simulink model "tensegrity_Val_like_sim_one_stage"  (R2022b)
settings: Solver=ode15s  StartTime=0.0  StopTime=10  MaxStep=0.001  RelTol=1e-3
InitFcn:
  | tensegrity_Val_like;
values from neighbouring files (symbols this model uses):
  a = 0.015    [parameters.m]
  A1 = [0.3, 0.3, 0.2]    [parameters_test_model.m]    (also in tensegrity_Val_like.m = [(G1+G2+G3)/3])
  bar_or_cable = 1    [parameters.m]
  bb = 100    [parameters.m]
  F1 = [pos1(1), pos1(2), pos1(3)]    [parameters.m]
  F2 = [pos1(1)+dist, pos1(2), pos1(3)]    [parameters.m]
  F3 = [pos1(1)+dist/2, pos1(2)+dist, pos1(3)]    [parameters.m]
  force_coefficient = -1    [parameters.m]
  kk = 5e4    (= 50000)    [parameters.m]
  l = [0.08 0.08 0.08 0.15]'    [parameters.m]
  lengths_0 = 0.9*lengths_0    [tensegrity_Val_like.m]
  lf = 0.05*ones(9, 1)    [parameters.m]
undefined symbols (not defined in the file or in its folder): X, Y, Z
libraries: nesl_utility x31, sm_lib x22
settings Model: Creator=zavrel  LastModifiedBy=zavrel

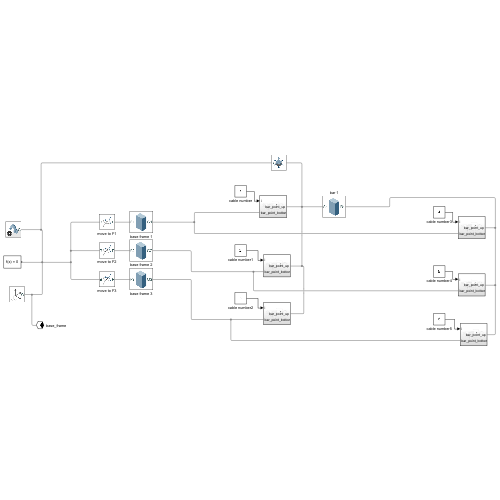
[thumbnail: Simulink's stored preview of the top-level diagram]
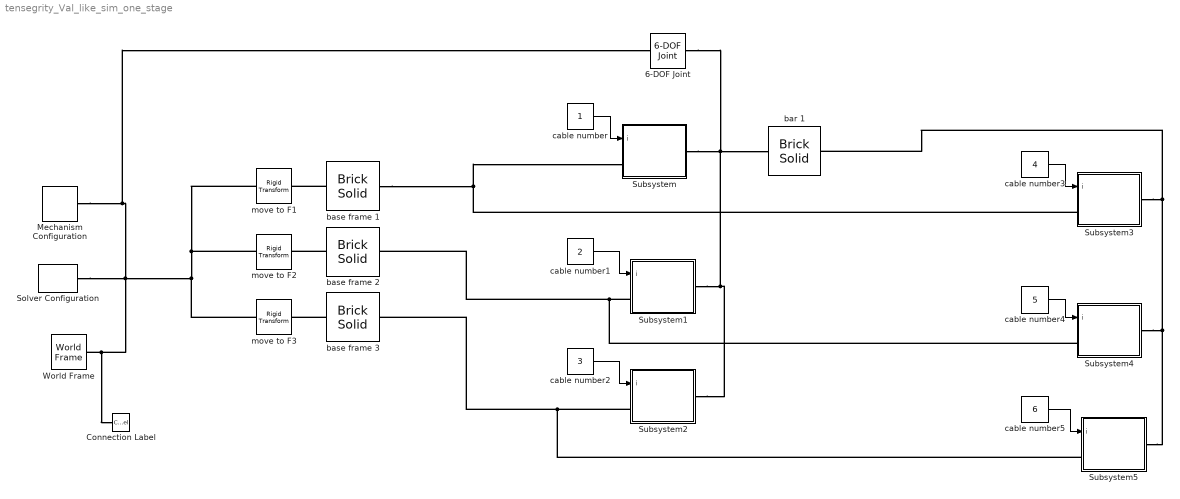
== system tensegrity_Val_like_sim_one_stage ==
  6-DOF Joint : sm_lib/Joints/6-DOF Joint  JointMode=Normal  SenseConstraintForce=off  SenseConstraintForceX=off  SenseConstraintForceY=off  SenseConstraintForceZ=off  SenseConstraintTorque=off  SenseConstraintTorqueX=off  SenseConstraintTorqueY=off  SenseConstraintTorqueZ=off  SenseTotalForce=off  SenseTotalForceX=off  SenseTotalForceY=off  SenseTotalForceZ=off  SenseTotalTorque=off  SenseTotalTorqueX=off  SenseTotalTorqueY=off  SenseTotalTorqueZ=off  CompositeWrenchDir=FollowerOnBase  CompositeWrenchFrame=BaseFrame  PxEquilibriumPosition=0  PxEquilibriumPositionUnits=m  PxSpringStiffness=0  PxSpringStiffnessUnits=N/m  PxDampingCoefficient=0  PxDampingCoefficientUnits=N/(m/s)  PxTorqueActuationMode=NoTorque  PxMotionActuationMode=ComputedMotion  PxSensePosition=off  PxSenseVelocity=off  PxSenseAcceleration=off  PxSenseTorqueForce=off  PxSenseLowerLimitTorqueForce=off  PxSenseUpperLimitTorqueForce=off  PxLowerLimitSpecify=off  PxLowerLimitBound=-1  PxLowerLimitBoundUnits=m  PxLowerLimitStiffness=1e6  PxLowerLimitStiffnessUnits=N/m  PxLowerLimitDamping=1e3  PxLowerLimitDampingUnits=N/(m/s)  PxLowerLimitTransitionRegionWidth=1e-4  PxLowerLimitTransitionRegionWidthUnits=m  PxUpperLimitSpecify=off  PxUpperLimitBound=1  PxUpperLimitBoundUnits=m  PxUpperLimitStiffness=1e6  PxUpperLimitStiffnessUnits=N/m  PxUpperLimitDamping=1e3  PxUpperLimitDampingUnits=N/(m/s)  PxUpperLimitTransitionRegionWidth=1e-4  PxUpperLimitTransitionRegionWidthUnits=m  PxPositionTargetSpecify=on  PxPositionTargetPriority=Low  PxPositionTargetValue=A1(1)  PxPositionTargetValueUnits=m  PxVelocityTargetSpecify=off  PxVelocityTargetPriority=High  PxVelocityTargetValue=0  PxVelocityTargetValueUnits=m/s  PyEquilibriumPosition=0  PyEquilibriumPositionUnits=m  PySpringStiffness=0  PySpringStiffnessUnits=N/m  PyDampingCoefficient=0  PyDampingCoefficientUnits=N/(m/s)  PyTorqueActuationMode=NoTorque  PyMotionActuationMode=ComputedMotion  PySensePosition=off  PySenseVelocity=off  PySenseAcceleration=off  PySenseTorqueForce=off  PySenseLowerLimitTorqueForce=off  PySenseUpperLimitTorqueForce=off  PyLowerLimitSpecify=off  PyLowerLimitBound=-1  PyLowerLimitBoundUnits=m  PyLowerLimitStiffness=1e6  PyLowerLimitStiffnessUnits=N/m  PyLowerLimitDamping=1e3  PyLowerLimitDampingUnits=N/(m/s)  PyLowerLimitTransitionRegionWidth=1e-4  PyLowerLimitTransitionRegionWidthUnits=m  PyUpperLimitSpecify=off  PyUpperLimitBound=1  PyUpperLimitBoundUnits=m  PyUpperLimitStiffness=1e6  PyUpperLimitStiffnessUnits=N/m  PyUpperLimitDamping=1e3  PyUpperLimitDampingUnits=N/(m/s)  PyUpperLimitTransitionRegionWidth=1e-4  PyUpperLimitTransitionRegionWidthUnits=m  PyPositionTargetSpecify=on  PyPositionTargetPriority=Low  PyPositionTargetValue=A1(2)  PyPositionTargetValueUnits=m  PyVelocityTargetSpecify=off  PyVelocityTargetPriority=High  PyVelocityTargetValue=0  PyVelocityTargetValueUnits=m/s  PzEquilibriumPosition=0  PzEquilibriumPositionUnits=m  PzSpringStiffness=0  PzSpringStiffnessUnits=N/m  PzDampingCoefficient=0  PzDampingCoefficientUnits=N/(m/s)  PzTorqueActuationMode=NoTorque  PzMotionActuationMode=ComputedMotion  PzSensePosition=off  PzSenseVelocity=off  PzSenseAcceleration=off  PzSenseTorqueForce=off  PzSenseLowerLimitTorqueForce=off  PzSenseUpperLimitTorqueForce=off  PzLowerLimitSpecify=off  PzLowerLimitBound=-1  PzLowerLimitBoundUnits=m  PzLowerLimitStiffness=1e6  PzLowerLimitStiffnessUnits=N/m  PzLowerLimitDamping=1e3  PzLowerLimitDampingUnits=N/(m/s)  PzLowerLimitTransitionRegionWidth=1e-4  PzLowerLimitTransitionRegionWidthUnits=m  PzUpperLimitSpecify=off  PzUpperLimitBound=1  PzUpperLimitBoundUnits=m  PzUpperLimitStiffness=1e6  PzUpperLimitStiffnessUnits=N/m  PzUpperLimitDamping=1e3  PzUpperLimitDampingUnits=N/(m/s)  PzUpperLimitTransitionRegionWidth=1e-4  PzUpperLimitTransitionRegionWidthUnits=m  PzPositionTargetSpecify=on  PzPositionTargetPriority=Low  PzPositionTargetValue=A1(3)  PzPositionTargetValueUnits=m  PzVelocityTargetSpecify=off  PzVelocityTargetPriority=High  PzVelocityTargetValue=0  PzVelocityTargetValueUnits=m/s  SphEqPosRotationMethod=None  SphEqPosRotationAngleUnits=deg  SphEqPosRotationStandardAxis=+Z  SphEqPosRotationAngle=0.0  SphEqPosRotationArbitraryAxis=[0 0 1]  SphEqPosFollAlignAxisA=+X  SphEqPosBaseAlignAxisA=+Y  SphEqPosFollAlignAxisB=+Y  SphEqPosBaseAlignAxisB=+Z  SphEqPosRotationSequenceAxes=FollowerAxes  SphEqPosRotationSequence=XYX  SphEqPosRotationSequenceAngles=[0 0 0]  SphEqPosRotationSequenceAnglesUnits=deg  SphEqPosRotationMatrix=[1 0 0; 0 1 0; 0 0 1]  SphEqPosQuaternion=[1 0 0 0]  SphSpringStiffness=0  SphSpringStiffnessUnits=N*m/deg  SphDampingCoefficient=0  SphDampingCoefficientUnits=N*m/(deg/s)  SphActuateTorqueX=off  SphActuateTorqueY=off  SphActuateTorqueZ=off  SphActuateTorque=off  SphTorqueActuationMode=NoTorque  SphMotionActuationMode=ComputedMotion  SphActuationFrame=BaseFrame  SphSensePosition=off  SphSenseVelocityX=off  SphSenseVelocityY=off  SphSenseVelocityZ=off  SphSenseVelocity=off  SphSenseAccelerationX=off  SphSenseAccelerationY=off  SphSenseAccelerationZ=off  SphSenseAcceleration=off  SphSenseTorqueX=off  SphSenseTorqueY=off  SphSenseTorqueZ=off  SphSenseTorqueForce=off  SphSenseLowerLimitTorqueMag=off  SphSenseUpperLimitTorqueMag=off  SphSensingFrame=BaseFrame  SphLowerLimitSpecify=off  SphLowerLimitBound=15  SphLowerLimitBoundUnits=deg  SphLowerLimitStiffness=1e4  SphLowerLimitStiffnessUnits=N*m/deg  SphLowerLimitDamping=10  SphLowerLimitDampingUnits=N*m/(deg/s)  SphLowerLimitTransitionRegionWidth=0.1  SphLowerLimitTransitionRegionWidthUnits=deg  SphUpperLimitSpecify=off  SphUpperLimitBound=45  SphUpperLimitBoundUnits=deg  SphUpperLimitStiffness=1e4  SphUpperLimitStiffnessUnits=N*m/deg  SphUpperLimitDamping=10  SphUpperLimitDampingUnits=N*m/(deg/s)  SphUpperLimitTransitionRegionWidth=0.1  SphUpperLimitTransitionRegionWidthUnits=deg  SphPositionTargetRotationMethod=None  SphPositionTargetRotationAngleUnits=deg  SphPositionTargetRotationStandardAxis=+Z  SphPositionTargetRotationAngle=0.0  SphPositionTargetRotationArbitraryAxis=[0 0 1]  SphPositionTargetFollAlignAxisA=+X  SphPositionTargetBaseAlignAxisA=+Y  SphPositionTargetFollAlignAxisB=+Y  SphPositionTargetBaseAlignAxisB=+Z  SphPositionTargetRotationSequenceAxes=FollowerAxes  SphPositionTargetRotationSequence=XYX  SphPositionTargetRotationSequenceAngles=[0 0 0]  SphPositionTargetRotationSequenceAnglesUnits=deg  SphPositionTargetRotationMatrix=[1 0 0; 0 1 0; 0 0 1]  SphPositionTargetQuaternion=[1 0 0 0]  SphPositionTargetSpecify=off  SphPositionTargetPriority=High  SphVelocityTargetValue=[0 0 0]  SphVelocityTargetValueUnits=deg/s  SphVelocityTargetSpecify=off  SphVelocityTargetPriority=High  SphVelocityTargetInFollowerFrame=on
  Connection Label : ConnectionLabel  Label=base_frame
  Mechanism Configuration : sm_lib/Utilities/Mechanism Configuration  UniformGravity=Constant  GravityVector=[0 0 -9.80665]  GravityUnits=m/s^2  LinearizationDelta=0.001  JointModeTransitionNonlinearIterations=2
  Solver Configuration : nesl_utility/Solver Configuration  PhysicalDomain=network_engine_domain  SubClassName=solver  LeftPortType=input  RightPortType=generic  Tones=[]  Harmonics=[]  SimulateNoise=off  Profile=off  UseLocalSampling=off  EnableSwitchedLinearOptims=on  FrequencyDomain=off  UseCCode=off  RelTol=0.001  AbsTol=0.001  MinStep=1e-09  ToWorkspace=off  RevertToSquareIcSolve=off  NumHomotopyIterations=100  PhasorMode=off  PhasorModeNumHarmonics=1  ConsistencySolver=NEWTON_XTOL_AFTER_FTOL  IndexReductionMethod=DerivativeReplacement  DoDC=off  ResidualTolerance=1e-09  ConsistencyTolSource=GLOBAL  ConsistencyAbsTol=0.001  ConsistencyRelTol=0.001  ConsistencyTolFactor=0.001  UseLocalSolver=off  LocalSolverChoice=NE_BACKWARD_EULER_ADVANCER  ResolveIndetEquations=on  FunctionEvalNumThread=1  LocalSolverSampleTime=0.001  DoFixedCost=off  MaxNonlinIter=3  MaxModeIter=2  ComputeImpulses=off  ImpulseIterations=2  LinearAlgebra=auto  LinearAlgebraNumThread=0  EquationFormulation=NE_TIME_EF  DelaysMemoryBudget=1024  AutomaticFiltering=on  FilteringTimeConstant=0.001  PartitionStorageMethod=AS_NEEDED  PartitionMemoryBudget=1024  PartitionMethod=ROBUST
  Subsystem : Subsystem
  Subsystem1 : Subsystem
  Subsystem2 : Subsystem
  Subsystem3 : Subsystem
  Subsystem4 : Subsystem
  Subsystem5 : Subsystem
  World Frame : sm_lib/Frames and Transforms/World Frame
  bar 1 : sm_lib/Body Elements/Brick Solid  GraphicAmbientColor=[0.15 0.15 0.15 1.0]  BasedOnType=Density  BrickDimensions=[a a l(1)]  BrickDimensionUnits=m  CenterOfMass=[0 0 0]  CenterOfMassUnits=m  GraphicDiffuseColor=[0.5 0.5 0.5]  Density=rho  DensityUnits=kg/m^3  DoExposeReferenceFrame=off  GraphicEmissiveColor=[0.0 0.0 0.0 1.0]  ExportEntireGeometry=off  SerializedFrames=<Frames><Frame><Id>Frame1</Id><Value><Name>A1</Name><Origin><Source>GeometricFeature</Source><FeatureName>-z surface</FeatureName></Origin><PrimaryAxis><DefinedDirection>+Z</DefinedDirection><Source>ReferenceFrame</Source><SourceDirection>+Z</SourceDirection><FeatureName></FeatureName></PrimaryAxis><SecondaryAxis><DefinedDirection>+X</DefinedDirection><Source>ReferenceFrame</Source><SourceDirection>+X</SourceDirection><FeatureName></FeatureName></SecondaryAxis></Value></Frame><Frame><Id>Frame2</Id><Value><Name>B1</Name><Origin><Source>GeometricFeature</Source><FeatureName>+z surface</FeatureName></Origin><PrimaryAxis><DefinedDirection>+Z</DefinedDirection><Source>ReferenceFrame</Source><SourceDirection>+Z</SourceDirection><FeatureName></FeatureName></PrimaryAxis><SecondaryAxis><DefinedDirection>+X</DefinedDirection><Source>ReferenceFrame</Source><SourceDirection>+X</SourceDirection><FeatureName></FeatureName></SecondaryAxis></Value></Frame></Frames>  MarkerShape=Sphere  MarkerSize=10  GraphicType=FromGeometry  InertiaType=CalculateFromGeometry  Mass=1  MassUnits=kg  MomentsOfInertia=[1 1 1]  MomentsOfInertiaUnits=kg*m^2  GraphicOpacity=1.0  ProductsOfInertia=[0 0 0]  ProductsOfInertiaUnits=kg*m^2  GraphicShininess=75  GraphicSpecularColor=[0.5 0.5 0.5 1.0]  GraphicVisPropType=SimpleVisualProperties
  base frame 1 : sm_lib/Body Elements/Brick Solid  GraphicAmbientColor=[0.15 0.15 0.15 1.0]  BasedOnType=Density  BrickDimensions=[a a lf(1)]  BrickDimensionUnits=m  CenterOfMass=[0 0 0]  CenterOfMassUnits=m  GraphicDiffuseColor=[0.5 0.5 0.5]  Density=rho  DensityUnits=kg/m^3  DoExposeReferenceFrame=off  GraphicEmissiveColor=[0.0 0.0 0.0 1.0]  ExportEntireGeometry=off  SerializedFrames=<Frames><Frame><Id>Frame1</Id><Value><Name>F1</Name><Origin><Source>GeometricFeature</Source><FeatureName>-z surface</FeatureName></Origin><PrimaryAxis><DefinedDirection>+Z</DefinedDirection><Source>ReferenceFrame</Source><SourceDirection>+Z</SourceDirection><FeatureName></FeatureName></PrimaryAxis><SecondaryAxis><DefinedDirection>+X</DefinedDirection><Source>ReferenceFrame</Source><SourceDirection>+X</SourceDirection><FeatureName></FeatureName></SecondaryAxis></Value></Frame><Frame><Id>Frame2</Id><Value><Name>G1</Name><Origin><Source>GeometricFeature</Source><FeatureName>+z surface</FeatureName></Origin><PrimaryAxis><DefinedDirection>+Z</DefinedDirection><Source>ReferenceFrame</Source><SourceDirection>+Z</SourceDirection><FeatureName></FeatureName></PrimaryAxis><SecondaryAxis><DefinedDirection>+X</DefinedDirection><Source>ReferenceFrame</Source><SourceDirection>+X</SourceDirection><FeatureName></FeatureName></SecondaryAxis></Value></Frame></Frames>  MarkerShape=Sphere  MarkerSize=10  GraphicType=FromGeometry  InertiaType=CalculateFromGeometry  Mass=1  MassUnits=kg  MomentsOfInertia=[1 1 1]  MomentsOfInertiaUnits=kg*m^2  GraphicOpacity=1.0  ProductsOfInertia=[0 0 0]  ProductsOfInertiaUnits=kg*m^2  GraphicShininess=75  GraphicSpecularColor=[0.5 0.5 0.5 1.0]  GraphicVisPropType=SimpleVisualProperties
  base frame 2 : sm_lib/Body Elements/Brick Solid  GraphicAmbientColor=[0.15 0.15 0.15 1.0]  BasedOnType=Density  BrickDimensions=[a a lf(2)]  BrickDimensionUnits=m  CenterOfMass=[0 0 0]  CenterOfMassUnits=m  GraphicDiffuseColor=[0.5 0.5 0.5]  Density=rho  DensityUnits=kg/m^3  DoExposeReferenceFrame=off  GraphicEmissiveColor=[0.0 0.0 0.0 1.0]  ExportEntireGeometry=off  SerializedFrames=<Frames><Frame><Id>Frame1</Id><Value><Name>F2</Name><Origin><Source>GeometricFeature</Source><FeatureName>-z surface</FeatureName></Origin><PrimaryAxis><DefinedDirection>+Z</DefinedDirection><Source>ReferenceFrame</Source><SourceDirection>+Z</SourceDirection><FeatureName></FeatureName></PrimaryAxis><SecondaryAxis><DefinedDirection>+X</DefinedDirection><Source>ReferenceFrame</Source><SourceDirection>+X</SourceDirection><FeatureName></FeatureName></SecondaryAxis></Value></Frame><Frame><Id>Frame2</Id><Value><Name>G2</Name><Origin><Source>GeometricFeature</Source><FeatureName>+z surface</FeatureName></Origin><PrimaryAxis><DefinedDirection>+Z</DefinedDirection><Source>ReferenceFrame</Source><SourceDirection>+Z</SourceDirection><FeatureName></FeatureName></PrimaryAxis><SecondaryAxis><DefinedDirection>+X</DefinedDirection><Source>ReferenceFrame</Source><SourceDirection>+X</SourceDirection><FeatureName></FeatureName></SecondaryAxis></Value></Frame></Frames>  MarkerShape=Sphere  MarkerSize=10  GraphicType=FromGeometry  InertiaType=CalculateFromGeometry  Mass=1  MassUnits=kg  MomentsOfInertia=[1 1 1]  MomentsOfInertiaUnits=kg*m^2  GraphicOpacity=1.0  ProductsOfInertia=[0 0 0]  ProductsOfInertiaUnits=kg*m^2  GraphicShininess=75  GraphicSpecularColor=[0.5 0.5 0.5 1.0]  GraphicVisPropType=SimpleVisualProperties
  base frame 3 : sm_lib/Body Elements/Brick Solid  GraphicAmbientColor=[0.15 0.15 0.15 1.0]  BasedOnType=Density  BrickDimensions=[a a lf(3)]  BrickDimensionUnits=m  CenterOfMass=[0 0 0]  CenterOfMassUnits=m  GraphicDiffuseColor=[0.5 0.5 0.5]  Density=rho  DensityUnits=kg/m^3  DoExposeReferenceFrame=off  GraphicEmissiveColor=[0.0 0.0 0.0 1.0]  ExportEntireGeometry=off  SerializedFrames=<Frames><Frame><Id>Frame1</Id><Value><Name>F3</Name><Origin><Source>GeometricFeature</Source><FeatureName>-z surface</FeatureName></Origin><PrimaryAxis><DefinedDirection>+Z</DefinedDirection><Source>ReferenceFrame</Source><SourceDirection>+Z</SourceDirection><FeatureName></FeatureName></PrimaryAxis><SecondaryAxis><DefinedDirection>+X</DefinedDirection><Source>ReferenceFrame</Source><SourceDirection>+X</SourceDirection><FeatureName></FeatureName></SecondaryAxis></Value></Frame><Frame><Id>Frame2</Id><Value><Name>G3</Name><Origin><Source>GeometricFeature</Source><FeatureName>+z surface</FeatureName></Origin><PrimaryAxis><DefinedDirection>+Z</DefinedDirection><Source>ReferenceFrame</Source><SourceDirection>+Z</SourceDirection><FeatureName></FeatureName></PrimaryAxis><SecondaryAxis><DefinedDirection>+X</DefinedDirection><Source>ReferenceFrame</Source><SourceDirection>+X</SourceDirection><FeatureName></FeatureName></SecondaryAxis></Value></Frame></Frames>  MarkerShape=Sphere  MarkerSize=10  GraphicType=FromGeometry  InertiaType=CalculateFromGeometry  Mass=1  MassUnits=kg  MomentsOfInertia=[1 1 1]  MomentsOfInertiaUnits=kg*m^2  GraphicOpacity=1.0  ProductsOfInertia=[0 0 0]  ProductsOfInertiaUnits=kg*m^2  GraphicShininess=75  GraphicSpecularColor=[0.5 0.5 0.5 1.0]  GraphicVisPropType=SimpleVisualProperties
  cable number : Constant
  cable number1 : Constant  Value=2
  cable number2 : Constant  Value=3
  cable number3 : Constant  Value=4
  cable number4 : Constant  Value=5
  cable number5 : Constant  Value=6
  move to F1 : sm_lib/Frames and Transforms/Rigid Transform  TranslationMethod=Cartesian  TranslationStandardOffset=0  TranslationLengthUnit=m  TranslationStandardAxis=+Z  TranslationCartesianOffset=[F1(1) F1(2) F1(3)]  TranslationROffset=0  TranslationROffsetUnits=m  TranslationZOffset=0  TranslationZOffsetUnits=m  TranslationThetaOffset=0  TranslationThetaOffsetUnits=deg  RotationMethod=None  RotationAngleUnits=deg  RotationStandardAxis=+Z  RotationAngle=0.0  RotationArbitraryAxis=[0 0 1]  FollAlignAxisA=+X  BaseAlignAxisA=+Y  FollAlignAxisB=+Y  BaseAlignAxisB=+Z  RotationSequenceAxes=FollowerAxes  RotationSequence=XYX  RotationSequenceAngles=[0 0 0]  RotationSequenceAnglesUnits=deg  RotationMatrix=[1 0 0; 0 1 0; 0 0 1]  Quaternion=[1 0 0 0]
  move to F2 : sm_lib/Frames and Transforms/Rigid Transform  TranslationMethod=Cartesian  TranslationStandardOffset=0  TranslationLengthUnit=m  TranslationStandardAxis=+Z  TranslationCartesianOffset=[F2(1) F2(2) F2(3)]  TranslationROffset=0  TranslationROffsetUnits=m  TranslationZOffset=0  TranslationZOffsetUnits=m  TranslationThetaOffset=0  TranslationThetaOffsetUnits=deg  RotationMethod=None  RotationAngleUnits=deg  RotationStandardAxis=+Z  RotationAngle=0.0  RotationArbitraryAxis=[0 0 1]  FollAlignAxisA=+X  BaseAlignAxisA=+Y  FollAlignAxisB=+Y  BaseAlignAxisB=+Z  RotationSequenceAxes=FollowerAxes  RotationSequence=XYX  RotationSequenceAngles=[0 0 0]  RotationSequenceAnglesUnits=deg  RotationMatrix=[1 0 0; 0 1 0; 0 0 1]  Quaternion=[1 0 0 0]
  move to F3 : sm_lib/Frames and Transforms/Rigid Transform  TranslationMethod=Cartesian  TranslationStandardOffset=0  TranslationLengthUnit=m  TranslationStandardAxis=+Z  TranslationCartesianOffset=[F3(1) F3(2) F3(3)]  TranslationROffset=0  TranslationROffsetUnits=m  TranslationZOffset=0  TranslationZOffsetUnits=m  TranslationThetaOffset=0  TranslationThetaOffsetUnits=deg  RotationMethod=None  RotationAngleUnits=deg  RotationStandardAxis=+Z  RotationAngle=0.0  RotationArbitraryAxis=[0 0 1]  FollAlignAxisA=+X  BaseAlignAxisA=+Y  FollAlignAxisB=+Y  BaseAlignAxisB=+Z  RotationSequenceAxes=FollowerAxes  RotationSequence=XYX  RotationSequenceAngles=[0 0 0]  RotationSequenceAnglesUnits=deg  RotationMatrix=[1 0 0; 0 1 0; 0 0 1]  Quaternion=[1 0 0 0]
  wires:
  cable number/1 -> Subsystem/1(i)
  cable number1/1 -> Subsystem1/1(i)
  cable number2/1 -> Subsystem2/1(i)
  cable number4/1 -> Subsystem4/1(i)
  cable number3/1 -> Subsystem3/1(i)
  cable number5/1 -> Subsystem5/1(i)
  connections:
  base frame 1/LConn1 -- move to F1/RConn1
  base frame 2/LConn1 -- move to F2/RConn1
  base frame 3/LConn1 -- move to F3/RConn1
  Mechanism Configuration/RConn1 -- 6-DOF Joint/LConn1 -- move to F3/LConn1 -- move to F2/LConn1 -- move to F1/LConn1 -- Connection Label/LConn1 -- World Frame/RConn1 -- Solver Configuration/RConn1
  Subsystem/RConn1 -- bar 1/LConn1 -- 6-DOF Joint/RConn1 -- Subsystem2/RConn1 -- Subsystem1/RConn1
  base frame 1/RConn1 -- Subsystem3/LConn1 -- Subsystem/LConn1
  base frame 2/RConn1 -- Subsystem4/LConn1 -- Subsystem1/LConn1
  base frame 3/RConn1 -- Subsystem5/LConn1 -- Subsystem2/LConn1
  Subsystem4/RConn1 -- Subsystem5/RConn1 -- Subsystem3/RConn1 -- bar 1/RConn1

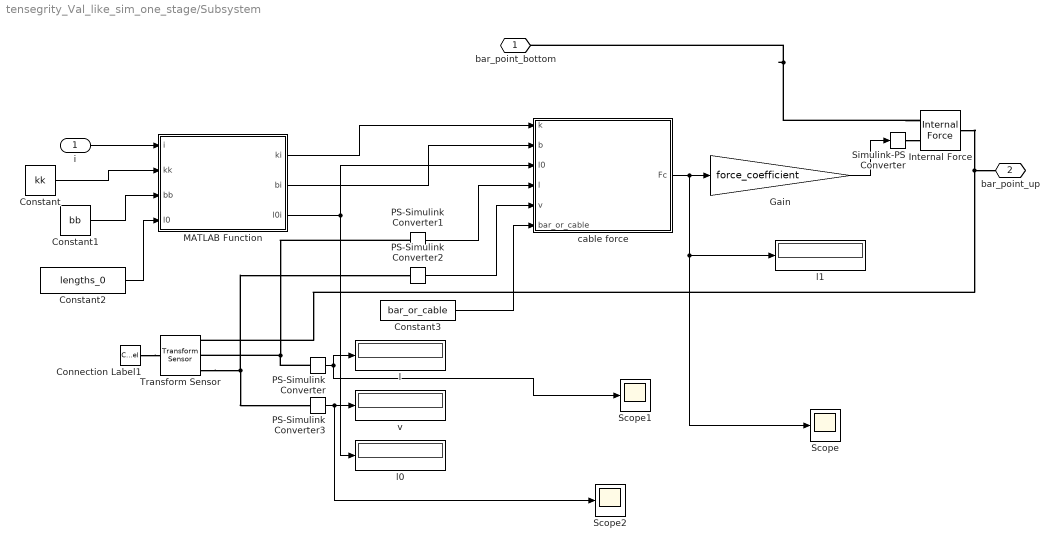
== system tensegrity_Val_like_sim_one_stage/Subsystem ==
  i : Inport
  Connection Label1 : ConnectionLabel  Label=base_frame
  Constant : Constant  Value=kk
  Constant1 : Constant  Value=bb
  Constant2 : Constant  Value=lengths_0
  Constant3 : Constant  Value=bar_or_cable
  Gain : Gain  Gain=force_coefficient
  Internal Force : sm_lib/Forces and Torques/Internal Force
  MATLAB Function : MATLAB Function  TreatAsAtomicUnit=on
  PS-Simulink Converter{,1..3} (4 alike) : nesl_utility/PS-Simulink Converter  PhysicalDomain=network_engine_domain  SubClassName=ps_output  LeftPortType=input  RightPortType=output  PseudoPeriodic=off  Frequencies=[]  VectorFormat=inherit  Unit=inherit  AffineConversion=off
  Scope : Scope
  Scope1 : Scope
  Scope2 : Scope
  Simulink-PS Converter : nesl_utility/Simulink-PS Converter  PhysicalDomain=network_engine_domain  SubClassName=ps_input  LeftPortType=input  RightPortType=output  PseudoPeriodic=off  Frequencies=[]  NoiseDistribution=none  NoiseParameters=[]  Unit=1  AffineConversion=off  FilteringAndDerivatives=provide  SimscapeFilterOrder=1  InputFilterTimeConstant=0.001  UdotUserProvided=0
  Transform Sensor : sm_lib/Frames and Transforms/Transform Sensor  MeasurementFrame=World  SenseAngle=off  SenseAxis=off  SenseQ=off  SenseR=off  SenseRotationSequence=off  RotationSequence=XYX  SenseOmegaX=off  SenseOmegaY=off  SenseOmegaZ=off  SenseQDot=off  SenseRDot=off  SenseAlphaX=off  SenseAlphaY=off  SenseAlphaZ=off  SenseQDDot=off  SenseRDDot=off  SenseX=off  SenseY=off  SenseZ=off  SenseRad=off  SenseAzim=off  SenseDist=on  SenseInc=off  SenseXDot=off  SenseYDot=off  SenseZDot=off  SenseRadDot=off  SenseAzimDot=off  SenseDistDot=on  SenseIncDot=off  SenseXDDot=off  SenseYDDot=off  SenseZDDot=off  SenseRadDDot=off  SenseAzimDDot=off  SenseDistDDot=off  SenseIncDDot=off
  cable force : MATLAB Function  TreatAsAtomicUnit=on
  l : Display
  l0 : Display
  l1 : Display
  v : Display
  bar_point_bottom : PMIOPort  Side=Left
  bar_point_up : PMIOPort  Port=2  Side=Right
  wires:
  cable force/1(Fc) -> Gain/1, Scope/1, l1/1
  PS-Simulink Converter/1 -> l/1, Scope1/1
  Constant2/1 -> MATLAB Function/4(l0)
  MATLAB Function/2(bi) -> cable force/2(b)
  Constant1/1 -> MATLAB Function/3(bb)
  Constant/1 -> MATLAB Function/2(kk)
  MATLAB Function/1(ki) -> cable force/1(k)
  PS-Simulink Converter1/1 -> cable force/4(l)
  MATLAB Function/3(l0i) -> l0/1, cable force/3(l0)
  i/1 -> MATLAB Function/1(i)
  Constant3/1 -> cable force/6(bar_or_cable)
  Gain/1 -> Simulink-PS Converter/1
  PS-Simulink Converter2/1 -> cable force/5(v)
  PS-Simulink Converter3/1 -> Scope2/1, v/1
  connections:
  Internal Force/LConn1 -- bar_point_bottom/RConn1
  PS-Simulink Converter/LConn1 -- PS-Simulink Converter1/LConn1 -- Transform Sensor/RConn2
  Simulink-PS Converter/RConn1 -- Internal Force/LConn2
  Internal Force/RConn1 -- bar_point_up/RConn1 -- Transform Sensor/RConn1
  Connection Label1/LConn1 -- Transform Sensor/LConn1
  Transform Sensor/RConn3 -- PS-Simulink Converter3/LConn1 -- PS-Simulink Converter2/LConn1

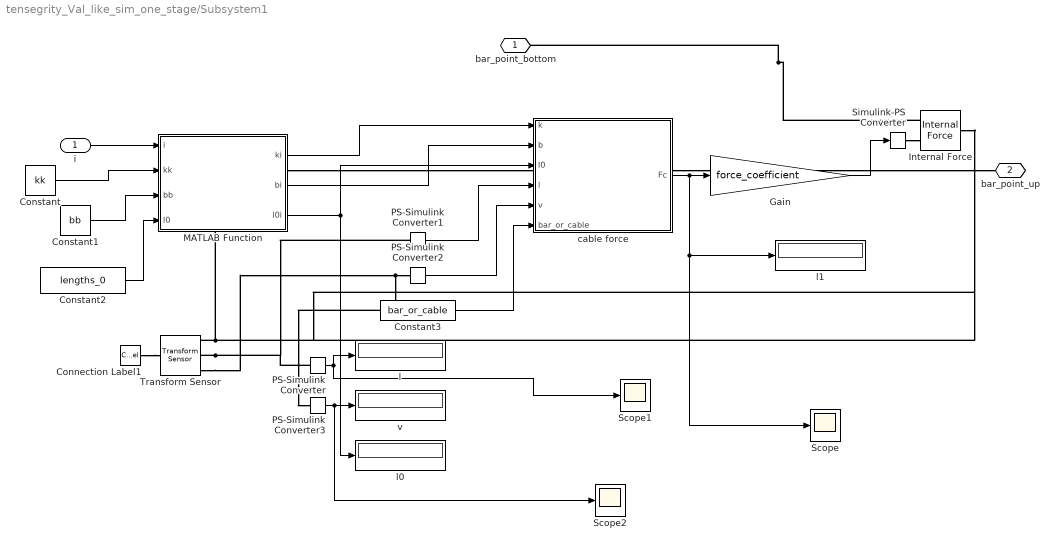
== system tensegrity_Val_like_sim_one_stage/Subsystem1 ==
  i : Inport
  Connection Label1 : ConnectionLabel  Label=base_frame
  Constant : Constant  Value=kk
  Constant1 : Constant  Value=bb
  Constant2 : Constant  Value=lengths_0
  Constant3 : Constant  Value=bar_or_cable
  Gain : Gain  Gain=force_coefficient
  Internal Force : sm_lib/Forces and Torques/Internal Force
  MATLAB Function : MATLAB Function  TreatAsAtomicUnit=on
  PS-Simulink Converter{,1..3} (4 alike) : nesl_utility/PS-Simulink Converter  PhysicalDomain=network_engine_domain  SubClassName=ps_output  LeftPortType=input  RightPortType=output  PseudoPeriodic=off  Frequencies=[]  VectorFormat=inherit  Unit=inherit  AffineConversion=off
  Scope : Scope
  Scope1 : Scope
  Scope2 : Scope
  Simulink-PS Converter : nesl_utility/Simulink-PS Converter  PhysicalDomain=network_engine_domain  SubClassName=ps_input  LeftPortType=input  RightPortType=output  PseudoPeriodic=off  Frequencies=[]  NoiseDistribution=none  NoiseParameters=[]  Unit=1  AffineConversion=off  FilteringAndDerivatives=provide  SimscapeFilterOrder=1  InputFilterTimeConstant=0.001  UdotUserProvided=0
  Transform Sensor : sm_lib/Frames and Transforms/Transform Sensor  MeasurementFrame=World  SenseAngle=off  SenseAxis=off  SenseQ=off  SenseR=off  SenseRotationSequence=off  RotationSequence=XYX  SenseOmegaX=off  SenseOmegaY=off  SenseOmegaZ=off  SenseQDot=off  SenseRDot=off  SenseAlphaX=off  SenseAlphaY=off  SenseAlphaZ=off  SenseQDDot=off  SenseRDDot=off  SenseX=off  SenseY=off  SenseZ=off  SenseRad=off  SenseAzim=off  SenseDist=on  SenseInc=off  SenseXDot=off  SenseYDot=off  SenseZDot=off  SenseRadDot=off  SenseAzimDot=off  SenseDistDot=on  SenseIncDot=off  SenseXDDot=off  SenseYDDot=off  SenseZDDot=off  SenseRadDDot=off  SenseAzimDDot=off  SenseDistDDot=off  SenseIncDDot=off
  cable force : MATLAB Function  TreatAsAtomicUnit=on
  l : Display
  l0 : Display
  l1 : Display
  v : Display
  bar_point_bottom : PMIOPort  Side=Left
  bar_point_up : PMIOPort  Port=2  Side=Right
  wires:
  PS-Simulink Converter3/1 -> v/1, Scope2/1
  PS-Simulink Converter2/1 -> cable force/5(v)
  Gain/1 -> Simulink-PS Converter/1
  Constant3/1 -> cable force/6(bar_or_cable)
  i/1 -> MATLAB Function/1(i)
  MATLAB Function/3(l0i) -> cable force/3(l0), l0/1
  PS-Simulink Converter1/1 -> cable force/4(l)
  MATLAB Function/1(ki) -> cable force/1(k)
  Constant/1 -> MATLAB Function/2(kk)
  Constant1/1 -> MATLAB Function/3(bb)
  MATLAB Function/2(bi) -> cable force/2(b)
  Constant2/1 -> MATLAB Function/4(l0)
  PS-Simulink Converter/1 -> Scope1/1, l/1
  cable force/1(Fc) -> l1/1, Scope/1, Gain/1
  connections:
  PS-Simulink Converter2/LConn1 -- PS-Simulink Converter3/LConn1 -- Transform Sensor/RConn3
  Connection Label1/LConn1 -- Transform Sensor/LConn1
  Transform Sensor/RConn1 -- bar_point_up/RConn1 -- Internal Force/RConn1
  Simulink-PS Converter/RConn1 -- Internal Force/LConn2
  Transform Sensor/RConn2 -- PS-Simulink Converter1/LConn1 -- PS-Simulink Converter/LConn1
  Internal Force/LConn1 -- bar_point_bottom/RConn1

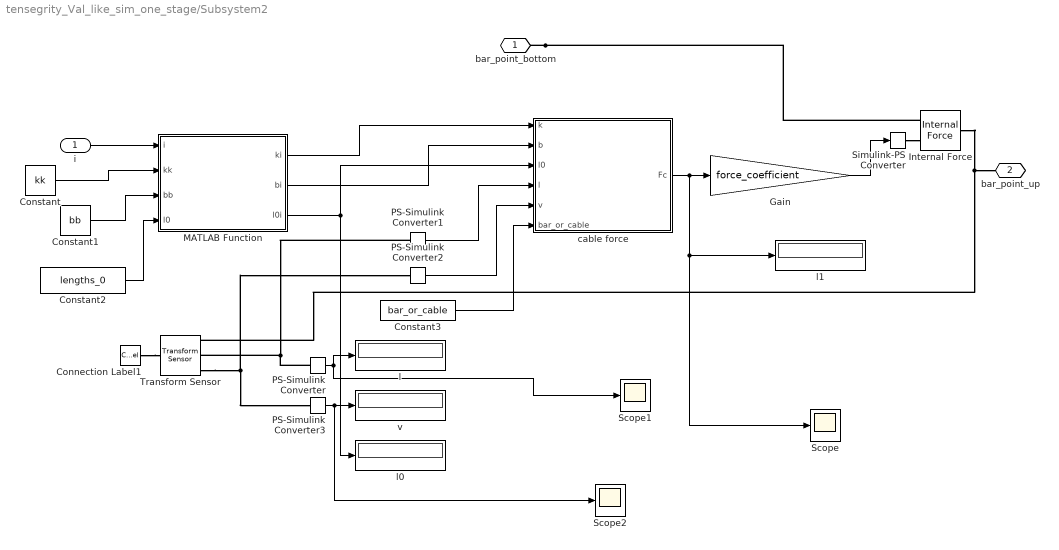
== system tensegrity_Val_like_sim_one_stage/Subsystem2 ==
  i : Inport
  Connection Label1 : ConnectionLabel  Label=base_frame
  Constant : Constant  Value=kk
  Constant1 : Constant  Value=bb
  Constant2 : Constant  Value=lengths_0
  Constant3 : Constant  Value=bar_or_cable
  Gain : Gain  Gain=force_coefficient
  Internal Force : sm_lib/Forces and Torques/Internal Force
  MATLAB Function : MATLAB Function  TreatAsAtomicUnit=on
  PS-Simulink Converter{,1..3} (4 alike) : nesl_utility/PS-Simulink Converter  PhysicalDomain=network_engine_domain  SubClassName=ps_output  LeftPortType=input  RightPortType=output  PseudoPeriodic=off  Frequencies=[]  VectorFormat=inherit  Unit=inherit  AffineConversion=off
  Scope : Scope
  Scope1 : Scope
  Scope2 : Scope
  Simulink-PS Converter : nesl_utility/Simulink-PS Converter  PhysicalDomain=network_engine_domain  SubClassName=ps_input  LeftPortType=input  RightPortType=output  PseudoPeriodic=off  Frequencies=[]  NoiseDistribution=none  NoiseParameters=[]  Unit=1  AffineConversion=off  FilteringAndDerivatives=provide  SimscapeFilterOrder=1  InputFilterTimeConstant=0.001  UdotUserProvided=0
  Transform Sensor : sm_lib/Frames and Transforms/Transform Sensor  MeasurementFrame=World  SenseAngle=off  SenseAxis=off  SenseQ=off  SenseR=off  SenseRotationSequence=off  RotationSequence=XYX  SenseOmegaX=off  SenseOmegaY=off  SenseOmegaZ=off  SenseQDot=off  SenseRDot=off  SenseAlphaX=off  SenseAlphaY=off  SenseAlphaZ=off  SenseQDDot=off  SenseRDDot=off  SenseX=off  SenseY=off  SenseZ=off  SenseRad=off  SenseAzim=off  SenseDist=on  SenseInc=off  SenseXDot=off  SenseYDot=off  SenseZDot=off  SenseRadDot=off  SenseAzimDot=off  SenseDistDot=on  SenseIncDot=off  SenseXDDot=off  SenseYDDot=off  SenseZDDot=off  SenseRadDDot=off  SenseAzimDDot=off  SenseDistDDot=off  SenseIncDDot=off
  cable force : MATLAB Function  TreatAsAtomicUnit=on
  l : Display
  l0 : Display
  l1 : Display
  v : Display
  bar_point_bottom : PMIOPort  Side=Left
  bar_point_up : PMIOPort  Port=2  Side=Right
  wires:
  cable force/1(Fc) -> Gain/1, Scope/1, l1/1
  PS-Simulink Converter/1 -> l/1, Scope1/1
  Constant2/1 -> MATLAB Function/4(l0)
  MATLAB Function/2(bi) -> cable force/2(b)
  Constant1/1 -> MATLAB Function/3(bb)
  Constant/1 -> MATLAB Function/2(kk)
  MATLAB Function/1(ki) -> cable force/1(k)
  PS-Simulink Converter1/1 -> cable force/4(l)
  MATLAB Function/3(l0i) -> l0/1, cable force/3(l0)
  i/1 -> MATLAB Function/1(i)
  Constant3/1 -> cable force/6(bar_or_cable)
  Gain/1 -> Simulink-PS Converter/1
  PS-Simulink Converter2/1 -> cable force/5(v)
  PS-Simulink Converter3/1 -> Scope2/1, v/1
  connections:
  bar_point_bottom/RConn1 -- Internal Force/LConn1
  PS-Simulink Converter/LConn1 -- PS-Simulink Converter1/LConn1 -- Transform Sensor/RConn2
  Simulink-PS Converter/RConn1 -- Internal Force/LConn2
  Internal Force/RConn1 -- bar_point_up/RConn1 -- Transform Sensor/RConn1
  Connection Label1/LConn1 -- Transform Sensor/LConn1
  Transform Sensor/RConn3 -- PS-Simulink Converter3/LConn1 -- PS-Simulink Converter2/LConn1

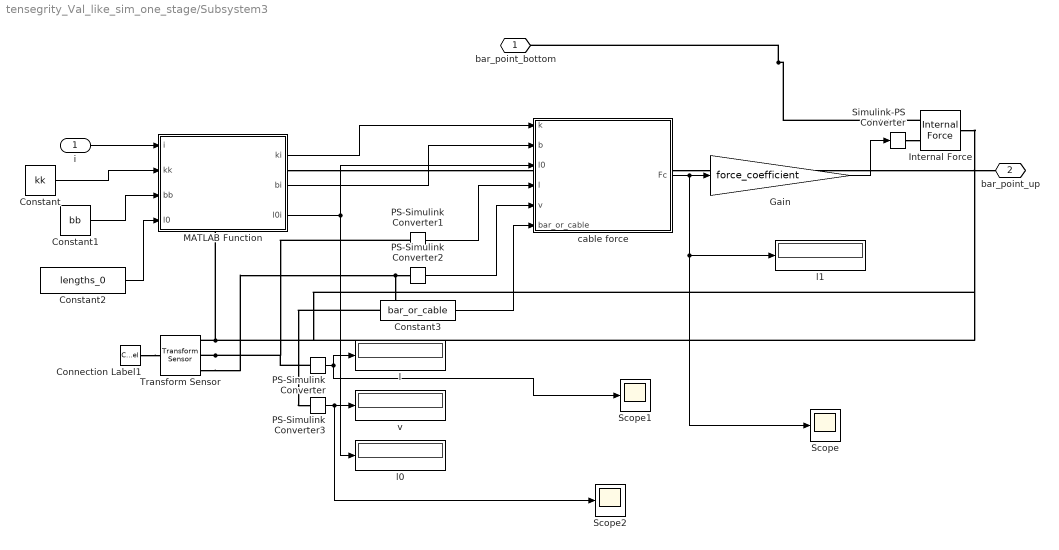
== system tensegrity_Val_like_sim_one_stage/Subsystem3 ==
  i : Inport
  Connection Label1 : ConnectionLabel  Label=base_frame
  Constant : Constant  Value=kk
  Constant1 : Constant  Value=bb
  Constant2 : Constant  Value=lengths_0
  Constant3 : Constant  Value=bar_or_cable
  Gain : Gain  Gain=force_coefficient
  Internal Force : sm_lib/Forces and Torques/Internal Force
  MATLAB Function : MATLAB Function  TreatAsAtomicUnit=on
  PS-Simulink Converter{,1..3} (4 alike) : nesl_utility/PS-Simulink Converter  PhysicalDomain=network_engine_domain  SubClassName=ps_output  LeftPortType=input  RightPortType=output  PseudoPeriodic=off  Frequencies=[]  VectorFormat=inherit  Unit=inherit  AffineConversion=off
  Scope : Scope
  Scope1 : Scope
  Scope2 : Scope
  Simulink-PS Converter : nesl_utility/Simulink-PS Converter  PhysicalDomain=network_engine_domain  SubClassName=ps_input  LeftPortType=input  RightPortType=output  PseudoPeriodic=off  Frequencies=[]  NoiseDistribution=none  NoiseParameters=[]  Unit=1  AffineConversion=off  FilteringAndDerivatives=provide  SimscapeFilterOrder=1  InputFilterTimeConstant=0.001  UdotUserProvided=0
  Transform Sensor : sm_lib/Frames and Transforms/Transform Sensor  MeasurementFrame=World  SenseAngle=off  SenseAxis=off  SenseQ=off  SenseR=off  SenseRotationSequence=off  RotationSequence=XYX  SenseOmegaX=off  SenseOmegaY=off  SenseOmegaZ=off  SenseQDot=off  SenseRDot=off  SenseAlphaX=off  SenseAlphaY=off  SenseAlphaZ=off  SenseQDDot=off  SenseRDDot=off  SenseX=off  SenseY=off  SenseZ=off  SenseRad=off  SenseAzim=off  SenseDist=on  SenseInc=off  SenseXDot=off  SenseYDot=off  SenseZDot=off  SenseRadDot=off  SenseAzimDot=off  SenseDistDot=on  SenseIncDot=off  SenseXDDot=off  SenseYDDot=off  SenseZDDot=off  SenseRadDDot=off  SenseAzimDDot=off  SenseDistDDot=off  SenseIncDDot=off
  cable force : MATLAB Function  TreatAsAtomicUnit=on
  l : Display
  l0 : Display
  l1 : Display
  v : Display
  bar_point_bottom : PMIOPort  Side=Left
  bar_point_up : PMIOPort  Port=2  Side=Right
  wires:
  PS-Simulink Converter3/1 -> v/1, Scope2/1
  PS-Simulink Converter2/1 -> cable force/5(v)
  Gain/1 -> Simulink-PS Converter/1
  Constant3/1 -> cable force/6(bar_or_cable)
  i/1 -> MATLAB Function/1(i)
  MATLAB Function/3(l0i) -> cable force/3(l0), l0/1
  PS-Simulink Converter1/1 -> cable force/4(l)
  MATLAB Function/1(ki) -> cable force/1(k)
  Constant/1 -> MATLAB Function/2(kk)
  Constant1/1 -> MATLAB Function/3(bb)
  MATLAB Function/2(bi) -> cable force/2(b)
  Constant2/1 -> MATLAB Function/4(l0)
  PS-Simulink Converter/1 -> Scope1/1, l/1
  cable force/1(Fc) -> l1/1, Scope/1, Gain/1
  connections:
  PS-Simulink Converter2/LConn1 -- PS-Simulink Converter3/LConn1 -- Transform Sensor/RConn3
  Connection Label1/LConn1 -- Transform Sensor/LConn1
  Transform Sensor/RConn1 -- bar_point_up/RConn1 -- Internal Force/RConn1
  Simulink-PS Converter/RConn1 -- Internal Force/LConn2
  Transform Sensor/RConn2 -- PS-Simulink Converter1/LConn1 -- PS-Simulink Converter/LConn1
  Internal Force/LConn1 -- bar_point_bottom/RConn1

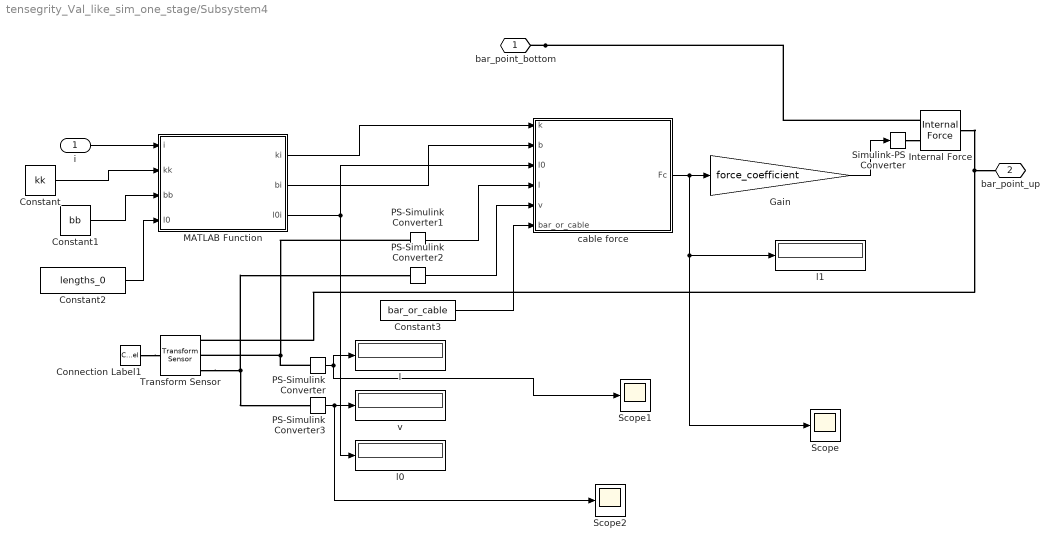
== system tensegrity_Val_like_sim_one_stage/Subsystem4 ==
  i : Inport
  Connection Label1 : ConnectionLabel  Label=base_frame
  Constant : Constant  Value=kk
  Constant1 : Constant  Value=bb
  Constant2 : Constant  Value=lengths_0
  Constant3 : Constant  Value=bar_or_cable
  Gain : Gain  Gain=force_coefficient
  Internal Force : sm_lib/Forces and Torques/Internal Force
  MATLAB Function : MATLAB Function  TreatAsAtomicUnit=on
  PS-Simulink Converter{,1..3} (4 alike) : nesl_utility/PS-Simulink Converter  PhysicalDomain=network_engine_domain  SubClassName=ps_output  LeftPortType=input  RightPortType=output  PseudoPeriodic=off  Frequencies=[]  VectorFormat=inherit  Unit=inherit  AffineConversion=off
  Scope : Scope
  Scope1 : Scope
  Scope2 : Scope
  Simulink-PS Converter : nesl_utility/Simulink-PS Converter  PhysicalDomain=network_engine_domain  SubClassName=ps_input  LeftPortType=input  RightPortType=output  PseudoPeriodic=off  Frequencies=[]  NoiseDistribution=none  NoiseParameters=[]  Unit=1  AffineConversion=off  FilteringAndDerivatives=provide  SimscapeFilterOrder=1  InputFilterTimeConstant=0.001  UdotUserProvided=0
  Transform Sensor : sm_lib/Frames and Transforms/Transform Sensor  MeasurementFrame=World  SenseAngle=off  SenseAxis=off  SenseQ=off  SenseR=off  SenseRotationSequence=off  RotationSequence=XYX  SenseOmegaX=off  SenseOmegaY=off  SenseOmegaZ=off  SenseQDot=off  SenseRDot=off  SenseAlphaX=off  SenseAlphaY=off  SenseAlphaZ=off  SenseQDDot=off  SenseRDDot=off  SenseX=off  SenseY=off  SenseZ=off  SenseRad=off  SenseAzim=off  SenseDist=on  SenseInc=off  SenseXDot=off  SenseYDot=off  SenseZDot=off  SenseRadDot=off  SenseAzimDot=off  SenseDistDot=on  SenseIncDot=off  SenseXDDot=off  SenseYDDot=off  SenseZDDot=off  SenseRadDDot=off  SenseAzimDDot=off  SenseDistDDot=off  SenseIncDDot=off
  cable force : MATLAB Function  TreatAsAtomicUnit=on
  l : Display
  l0 : Display
  l1 : Display
  v : Display
  bar_point_bottom : PMIOPort  Side=Left
  bar_point_up : PMIOPort  Port=2  Side=Right
  wires:
  cable force/1(Fc) -> Gain/1, Scope/1, l1/1
  PS-Simulink Converter/1 -> l/1, Scope1/1
  Constant2/1 -> MATLAB Function/4(l0)
  MATLAB Function/2(bi) -> cable force/2(b)
  Constant1/1 -> MATLAB Function/3(bb)
  Constant/1 -> MATLAB Function/2(kk)
  MATLAB Function/1(ki) -> cable force/1(k)
  PS-Simulink Converter1/1 -> cable force/4(l)
  MATLAB Function/3(l0i) -> l0/1, cable force/3(l0)
  i/1 -> MATLAB Function/1(i)
  Constant3/1 -> cable force/6(bar_or_cable)
  Gain/1 -> Simulink-PS Converter/1
  PS-Simulink Converter2/1 -> cable force/5(v)
  PS-Simulink Converter3/1 -> Scope2/1, v/1
  connections:
  bar_point_bottom/RConn1 -- Internal Force/LConn1
  PS-Simulink Converter/LConn1 -- PS-Simulink Converter1/LConn1 -- Transform Sensor/RConn2
  Simulink-PS Converter/RConn1 -- Internal Force/LConn2
  Internal Force/RConn1 -- bar_point_up/RConn1 -- Transform Sensor/RConn1
  Connection Label1/LConn1 -- Transform Sensor/LConn1
  Transform Sensor/RConn3 -- PS-Simulink Converter3/LConn1 -- PS-Simulink Converter2/LConn1

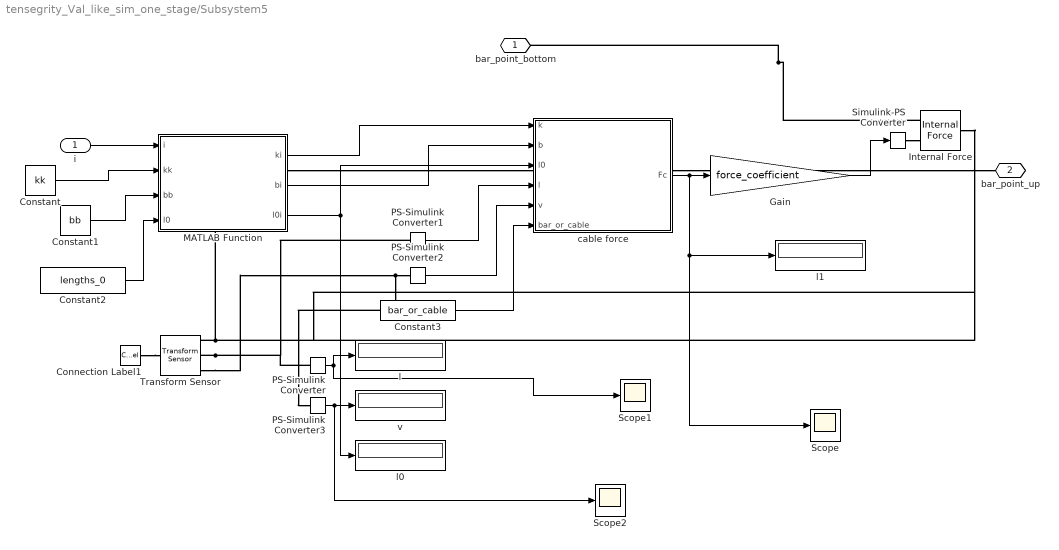
== system tensegrity_Val_like_sim_one_stage/Subsystem5 ==
  i : Inport
  Connection Label1 : ConnectionLabel  Label=base_frame
  Constant : Constant  Value=kk
  Constant1 : Constant  Value=bb
  Constant2 : Constant  Value=lengths_0
  Constant3 : Constant  Value=bar_or_cable
  Gain : Gain  Gain=force_coefficient
  Internal Force : sm_lib/Forces and Torques/Internal Force
  MATLAB Function : MATLAB Function  TreatAsAtomicUnit=on
  PS-Simulink Converter{,1..3} (4 alike) : nesl_utility/PS-Simulink Converter  PhysicalDomain=network_engine_domain  SubClassName=ps_output  LeftPortType=input  RightPortType=output  PseudoPeriodic=off  Frequencies=[]  VectorFormat=inherit  Unit=inherit  AffineConversion=off
  Scope : Scope
  Scope1 : Scope
  Scope2 : Scope
  Simulink-PS Converter : nesl_utility/Simulink-PS Converter  PhysicalDomain=network_engine_domain  SubClassName=ps_input  LeftPortType=input  RightPortType=output  PseudoPeriodic=off  Frequencies=[]  NoiseDistribution=none  NoiseParameters=[]  Unit=1  AffineConversion=off  FilteringAndDerivatives=provide  SimscapeFilterOrder=1  InputFilterTimeConstant=0.001  UdotUserProvided=0
  Transform Sensor : sm_lib/Frames and Transforms/Transform Sensor  MeasurementFrame=World  SenseAngle=off  SenseAxis=off  SenseQ=off  SenseR=off  SenseRotationSequence=off  RotationSequence=XYX  SenseOmegaX=off  SenseOmegaY=off  SenseOmegaZ=off  SenseQDot=off  SenseRDot=off  SenseAlphaX=off  SenseAlphaY=off  SenseAlphaZ=off  SenseQDDot=off  SenseRDDot=off  SenseX=off  SenseY=off  SenseZ=off  SenseRad=off  SenseAzim=off  SenseDist=on  SenseInc=off  SenseXDot=off  SenseYDot=off  SenseZDot=off  SenseRadDot=off  SenseAzimDot=off  SenseDistDot=on  SenseIncDot=off  SenseXDDot=off  SenseYDDot=off  SenseZDDot=off  SenseRadDDot=off  SenseAzimDDot=off  SenseDistDDot=off  SenseIncDDot=off
  cable force : MATLAB Function  TreatAsAtomicUnit=on
  l : Display
  l0 : Display
  l1 : Display
  v : Display
  bar_point_bottom : PMIOPort  Side=Left
  bar_point_up : PMIOPort  Port=2  Side=Right
  wires:
  PS-Simulink Converter3/1 -> v/1, Scope2/1
  PS-Simulink Converter2/1 -> cable force/5(v)
  Gain/1 -> Simulink-PS Converter/1
  Constant3/1 -> cable force/6(bar_or_cable)
  i/1 -> MATLAB Function/1(i)
  MATLAB Function/3(l0i) -> cable force/3(l0), l0/1
  PS-Simulink Converter1/1 -> cable force/4(l)
  MATLAB Function/1(ki) -> cable force/1(k)
  Constant/1 -> MATLAB Function/2(kk)
  Constant1/1 -> MATLAB Function/3(bb)
  MATLAB Function/2(bi) -> cable force/2(b)
  Constant2/1 -> MATLAB Function/4(l0)
  PS-Simulink Converter/1 -> Scope1/1, l/1
  cable force/1(Fc) -> l1/1, Scope/1, Gain/1
  connections:
  PS-Simulink Converter2/LConn1 -- PS-Simulink Converter3/LConn1 -- Transform Sensor/RConn3
  Connection Label1/LConn1 -- Transform Sensor/LConn1
  Transform Sensor/RConn1 -- bar_point_up/RConn1 -- Internal Force/RConn1
  Simulink-PS Converter/RConn1 -- Internal Force/LConn2
  Transform Sensor/RConn2 -- PS-Simulink Converter1/LConn1 -- PS-Simulink Converter/LConn1
  Internal Force/LConn1 -- bar_point_bottom/RConn1

== matlab function tensegrity_Val_like_sim_one_stage/Subsystem4/MATLAB Function ==
  data: i input; ki output; kk input; bb input; l0 input; bi output; l0i output
function [ki, bi, l0i] = parameter_selection(i, kk, bb, l0)

l0i=l0(i);
ki=kk;
bi=bb;

== matlab function tensegrity_Val_like_sim_one_stage/Subsystem/MATLAB Function ==
  data: i input; ki output; kk input; bb input; l0 input; bi output; l0i output
function [ki, bi, l0i] = parameter_selection(i, kk, bb, l0)

l0i=l0(i);
ki=kk;
bi=bb;

== matlab function tensegrity_Val_like_sim_one_stage/Subsystem4/cable force ==
  data: k input; Fc output; b input; l0 input; l input; v input; bar_or_cable input
function Fc = fcn(k, b, l0, l, v, bar_or_cable)

Fc=0; %if not bar, but cable only

if(l>l0)
  Fc=k*(l-l0) - b*v;
end;

if(bar_or_cable==1) % if bar==1, the force can act in both directions
  Fc=k*(l-l0) - b*v;
end;

== matlab function tensegrity_Val_like_sim_one_stage/Subsystem5/MATLAB Function ==
  data: i input; ki output; kk input; bb input; l0 input; bi output; l0i output
function [ki, bi, l0i] = parameter_selection(i, kk, bb, l0)

l0i=l0(i);
ki=kk;
bi=bb;

== matlab function tensegrity_Val_like_sim_one_stage/Subsystem5/cable force ==
  data: k input; Fc output; b input; l0 input; l input; v input; bar_or_cable input
function Fc = fcn(k, b, l0, l, v, bar_or_cable)

Fc=0; %if not bar, but cable only

if(l>l0)
  Fc=k*(l-l0) - b*v;
end;

if(bar_or_cable==1) % if bar==1, the force can act in both directions
  Fc=k*(l-l0) - b*v;
end;

== matlab function tensegrity_Val_like_sim_one_stage/Subsystem/cable force ==
  data: k input; Fc output; b input; l0 input; l input; v input; bar_or_cable input
function Fc = fcn(k, b, l0, l, v, bar_or_cable)

Fc=0; %if not bar, but cable only

if(l>l0)
  Fc=k*(l-l0) - b*v;
end;

if(bar_or_cable==1) % if bar==1, the force can act in both directions
  Fc=k*(l-l0) - b*v;
end;

== matlab function tensegrity_Val_like_sim_one_stage/Subsystem1/MATLAB Function ==
  data: i input; ki output; kk input; bb input; l0 input; bi output; l0i output
function [ki, bi, l0i] = parameter_selection(i, kk, bb, l0)

l0i=l0(i);
ki=kk;
bi=bb;

== matlab function tensegrity_Val_like_sim_one_stage/Subsystem1/cable force ==
  data: k input; Fc output; b input; l0 input; l input; v input; bar_or_cable input
function Fc = fcn(k, b, l0, l, v, bar_or_cable)

Fc=0; %if not bar, but cable only

if(l>l0)
  Fc=k*(l-l0) - b*v;
end;

if(bar_or_cable==1) % if bar==1, the force can act in both directions
  Fc=k*(l-l0) - b*v;
end;

== matlab function tensegrity_Val_like_sim_one_stage/Subsystem2/MATLAB Function ==
  data: i input; ki output; kk input; bb input; l0 input; bi output; l0i output
function [ki, bi, l0i] = parameter_selection(i, kk, bb, l0)

l0i=l0(i);
ki=kk;
bi=bb;

== matlab function tensegrity_Val_like_sim_one_stage/Subsystem2/cable force ==
  data: k input; Fc output; b input; l0 input; l input; v input; bar_or_cable input
function Fc = fcn(k, b, l0, l, v, bar_or_cable)

Fc=0; %if not bar, but cable only

if(l>l0)
  Fc=k*(l-l0) - b*v;
end;

if(bar_or_cable==1) % if bar==1, the force can act in both directions
  Fc=k*(l-l0) - b*v;
end;

== matlab function tensegrity_Val_like_sim_one_stage/Subsystem3/MATLAB Function ==
  data: i input; ki output; kk input; bb input; l0 input; bi output; l0i output
function [ki, bi, l0i] = parameter_selection(i, kk, bb, l0)

l0i=l0(i);
ki=kk;
bi=bb;

== matlab function tensegrity_Val_like_sim_one_stage/Subsystem3/cable force ==
  data: k input; Fc output; b input; l0 input; l input; v input; bar_or_cable input
function Fc = fcn(k, b, l0, l, v, bar_or_cable)

Fc=0; %if not bar, but cable only

if(l>l0)
  Fc=k*(l-l0) - b*v;
end;

if(bar_or_cable==1) % if bar==1, the force can act in both directions
  Fc=k*(l-l0) - b*v;
end;
